simulink model "Direct_PyTorchExportedProgra"  (R2026a)
settings: Solver=FixedStepAuto  StopTime=16.5  FixedStep=1.5  EnableMultiTasking=on
libraries: dlosslib x1
settings Model: ExtModeTrigDuration=2  Creator=hravisha  LastModifiedBy=hravisha
settings SolverCC: PositivePriorityOrder=on
settings OptimizationCC: MaxStackSize=200000
settings HardwareCC: ProdLargestAtomicInteger=Long  ProdLargestAtomicFloat=Double  ProdHWDeviceType=ARM Compatible->ARM Cortex-A (32-bit)
settings ModelReferenceCC: PropagateVarSize=During execution
settings RTWCC: SystemTargetFile=ert.tlc  HardwareBoard=Raspberry Pi  TLCOptions="-aInlineSetEventsForThisBaseRateFcn=TLC_FALSE -aSuppressMultiTaskScheduler=TLC_FALSE  -aRateBasedStepFcn=0"  Toolchain=GNU GCC RPIUtils  BuildConfiguration=Faster Runs  Description=Embedded Coder
settings ERTTargetCC: ExtModeTransport=2.0  SupportVariableSizeSignals=on

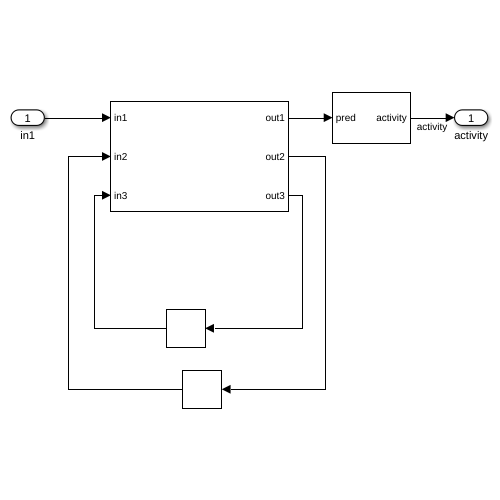
[thumbnail: Simulink's stored preview of the top-level diagram]
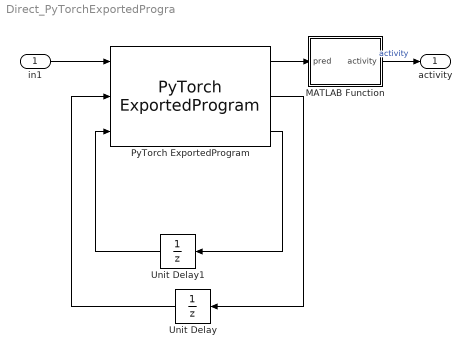
== system Direct_PyTorchExportedProgra ==
  in1 : Inport  OutDataTypeStr=single  PortDimensions=[1 75 3]  SampleTime=[1.5,0]
  MATLAB Function : MATLAB Function  TreatAsAtomicUnit=on
  PyTorch ExportedProgram : dlosslib/PyTorch ExportedProgram  ModelFilePath=/local-ssd/hravisha/directCodegenLectureSeminar/matlab_demo/stateful_lstm.pt2  SampleTime=-1  InputsTable={ 'in1', 'single', '[1 75 3]', '[1 2 3]'; 'in2', 'single', '[1 1 50]', '[1 2 3]'; 'in3', 'single', '[1 1 50]', '[1 2 3]' }  OutputsTable={ 'out1', 'single', '[1 75 5]', '[1 75 5]', '[1 2 3]'; 'out2', 'single', '[1 1 50]', '[1 1 50]', '[1 2 3]'; 'out3', 'single', '[1 1 50]', '[1 1 50]', '[1 2 3]' }  LastKnownModelFilePath=/local-ssd/hravisha/directCodegenLectureSeminar/matlab_demo/stateful_lstm.pt2  LastKnownModelTimeStamp=740076.3848379629  LastKnownFcnName=<empty>
  Unit Delay : UnitDelay  InitialCondition=zeros(1,1,50,'single')  SampleTime=-1
  Unit Delay1 : UnitDelay  InitialCondition=zeros(1,1,50,'single')  SampleTime=-1
  activity : Outport  OutDataTypeStr=Enum: ActivityLabel  PortDimensions=1  SampleTime=[1.5,0]
  wires:
  MATLAB Function/1(activity) -> activity/1  "activity"
  PyTorch ExportedProgram/3 -> Unit Delay1/1
  PyTorch ExportedProgram/2 -> Unit Delay/1
  PyTorch ExportedProgram/1 -> MATLAB Function/1(pred)
  in1/1 -> PyTorch ExportedProgram/1
  Unit Delay1/1 -> PyTorch ExportedProgram/3
  Unit Delay/1 -> PyTorch ExportedProgram/2

== matlab function Direct_PyTorchExportedProgra/MATLAB Function ==
  data: pred input; activity output
function activity = classifyActivity(pred)
    % pred is [1, 75, 5] — take last timestep, find argmax
    lastStep = pred(1, end, :);       % [1, 1, 5]
    scores = squeeze(lastStep);        % [5, 1]
    [~, idx] = max(scores);
    activity = ActivityLabel(idx);
end
